simulink model "IMU_Filtering"  (R2021a)
settings: Solver=ode1  StartTime=0.0  StopTime=t_tot  FixedStep=T  RelTol=1e-3
values from neighbouring files (symbols this model uses):
  acc_init_matrix = [acc_init_matrix_1; acc_init_matrix_2]    [Main_Filtering.m]
  calibration_flag = calibration_flag+1    (= 1)    [Main_Filtering.m]
  chain_id_matrix = [little_chain ... (first row only)    [Main_Filtering.m]
  filter_par_vec = [beta, sample_f, max_acc_norm, min_acc_norm, gyro_th,                     n_imus, n_orientations, n_chains, n_phalanges]    [Main_Filtering.m]
  q_init_matrix = q_matrix.data(:,:,end)    [Main_Filtering.m]
  q_off_matrix = q_matrix.data(:,:,end)    [Main_Filtering.m]
undefined symbols (not defined in the file or in its folder): deg, s
libraries: CP_library x1, QB_pacer_lib x1, qbmove_library x1
settings Model: Creator=murad  LastModifiedBy=sohei
settings SolverCC: AlgebraicLoopSolver=TrustRegion
settings DataIOCC: ReturnWorkspaceOutputs=off
settings DebuggingCC: SFMachineParentedDataDiag=warning  ArithmeticOperatorsInVariantConditions=warning
settings SFSimCC: CustomCodeUndefinedFunction=UseInterfaceOnly

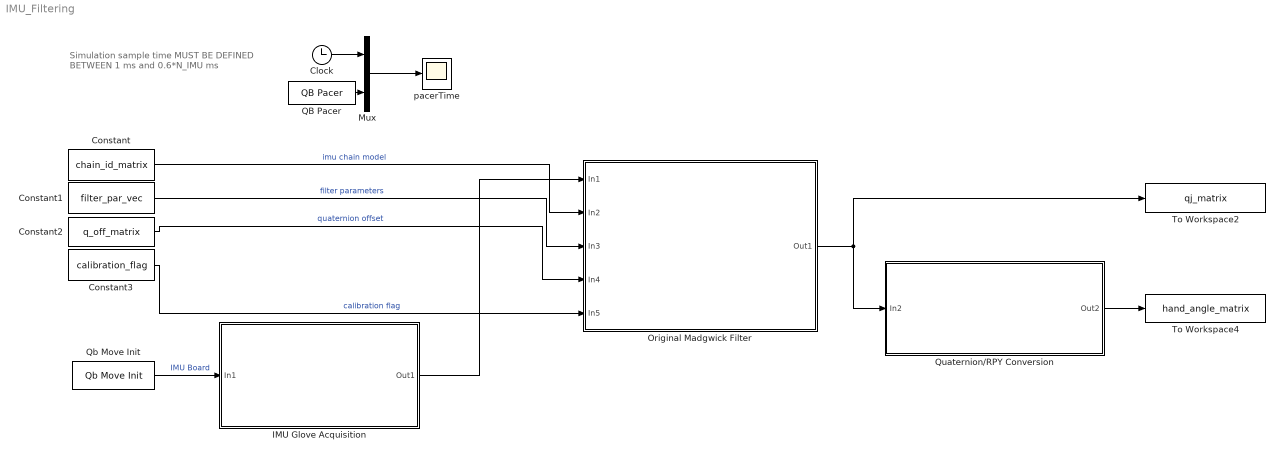
== system IMU_Filtering ==
  note: Simulation sample time
      | MUST BE DEFINED BETWEEN
      | 1 ms and 0.6*N_IMU ms
  Clock : Clock
  Constant : Constant  Value=chain_id_matrix
  Constant1 : Constant  Value=filter_par_vec
  Constant2 : Constant  Value=q_off_matrix
  Constant3 : Constant  Value=calibration_flag
  IMU Glove Acquisition : Subsystem
  Mux : Mux  Inputs=2
  Original Madgwick Filter : Subsystem
  QB Pacer : QB_pacer_lib/QB Pacer  simTimePerRealTime=1
      settings: SourceProductName=QB Pacer
  Qb Move Init : qbmove_library/Qb Move Init  NUMBER_OF_COM='COM3'  BAUD_RATE_COM=2000000
      settings: SourceProductName=Qb Move Library
  Quaternion/RPY Conversion : Subsystem
  To Workspace2 : ToWorkspace  VariableName=qj_matrix  SaveFormat=Timeseries  SampleTime=-1
  To Workspace4 : ToWorkspace  VariableName=hand_angle_matrix  SaveFormat=Timeseries  SampleTime=-1
  pacerTime : Scope
  wires:
  Mux/1 -> pacerTime/1
  QB Pacer/1 -> Mux/2
  Clock/1 -> Mux/1
  Qb Move Init/1 -> IMU Glove Acquisition/1(In1)  "IMU Board"
  IMU Glove Acquisition/1(Out1) -> Original Madgwick Filter/1(In1)
  Original Madgwick Filter/1(Out1) -> To Workspace2/1, Quaternion/RPY Conversion/1(In2)
  Quaternion/RPY Conversion/1(Out2) -> To Workspace4/1
  Constant/1 -> Original Madgwick Filter/2(In2)  "imu chain model"
  Constant1/1 -> Original Madgwick Filter/3(In3)  "filter parameters"
  Constant2/1 -> Original Madgwick Filter/4(In4)  "quaternion offset"
  Constant3/1 -> Original Madgwick Filter/5(In5)  "calibration flag"

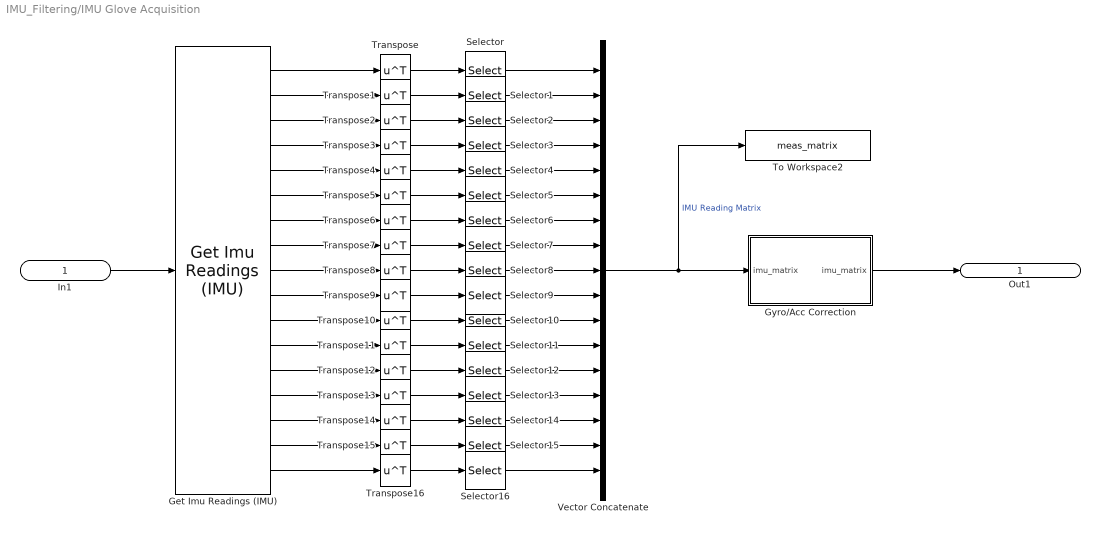
== system IMU_Filtering/IMU Glove Acquisition ==
  In1 : Inport
  Get Imu Readings (IMU) : CP_library/Get Imu Readings (IMU)  ID=3  N_IMU=17  DAISY_CHAINING=off  ACC_UNITY=G  GYRO_UNITY=deg/s  MAG_UNITY=uT
      settings: SourceProductName=Centro Piaggio Library
  Gyro/Acc Correction : MATLAB Function  TreatAsAtomicUnit=on
  Selector{,1..16} (17 alike) : Selector  InputPortWidth=14  IndexOptions=Index vector (dialog)  Indices=[1 2 3 4 5 6]  OutputSizes=1
  To Workspace2 : ToWorkspace  VariableName=meas_matrix  SaveFormat=Timeseries  SampleTime=-1
  Transpose{,1..16} (17 alike) : Math  Operator=transpose  SignedPower=on  SaturateOnIntegerOverflow=on
  Vector Concatenate : Concatenate  NumInputs=17  Mode=Multidimensional array  ConcatenateDimension=2
  Out1 : Outport  VectorParamsAs1DForOutWhenUnconnected=off
  wires:
  Get Imu Readings (IMU)/4 -> Transpose3/1
  Get Imu Readings (IMU)/3 -> Transpose2/1
  Transpose15/1 -> Selector15/1
  Transpose14/1 -> Selector14/1
  Transpose11/1 -> Selector11/1
  Get Imu Readings (IMU)/10 -> Transpose9/1
  Get Imu Readings (IMU)/8 -> Transpose7/1
  Get Imu Readings (IMU)/14 -> Transpose13/1
  Transpose7/1 -> Selector7/1
  Get Imu Readings (IMU)/7 -> Transpose6/1
  Transpose13/1 -> Selector13/1
  Get Imu Readings (IMU)/2 -> Transpose1/1
  Transpose6/1 -> Selector6/1
  In1/1 -> Get Imu Readings (IMU)/1
  Selector6/1 -> Vector Concatenate/7
  Selector4/1 -> Vector Concatenate/5
  Selector10/1 -> Vector Concatenate/11
  Transpose2/1 -> Selector2/1
  Selector9/1 -> Vector Concatenate/10
  Transpose9/1 -> Selector9/1
  Get Imu Readings (IMU)/13 -> Transpose12/1
  Selector5/1 -> Vector Concatenate/6
  Selector3/1 -> Vector Concatenate/4
  Get Imu Readings (IMU)/12 -> Transpose11/1
  Get Imu Readings (IMU)/16 -> Transpose15/1
  Get Imu Readings (IMU)/11 -> Transpose10/1
  Selector8/1 -> Vector Concatenate/9
  Get Imu Readings (IMU)/9 -> Transpose8/1
  Selector1/1 -> Vector Concatenate/2
  Transpose/1 -> Selector/1
  Get Imu Readings (IMU)/5 -> Transpose4/1
  Selector2/1 -> Vector Concatenate/3
  Selector14/1 -> Vector Concatenate/15
  Selector7/1 -> Vector Concatenate/8
  Transpose1/1 -> Selector1/1
  Get Imu Readings (IMU)/15 -> Transpose14/1
  Selector11/1 -> Vector Concatenate/12
  Get Imu Readings (IMU)/6 -> Transpose5/1
  Selector13/1 -> Vector Concatenate/14
  Selector16/1 -> Vector Concatenate/17
  Transpose5/1 -> Selector5/1
  Transpose3/1 -> Selector3/1
  Transpose10/1 -> Selector10/1
  Selector12/1 -> Vector Concatenate/13
  Selector15/1 -> Vector Concatenate/16
  Transpose4/1 -> Selector4/1
  Get Imu Readings (IMU)/17 -> Transpose16/1
  Transpose8/1 -> Selector8/1
  Selector/1 -> Vector Concatenate/1
  Get Imu Readings (IMU)/1 -> Transpose/1
  Vector Concatenate/1 -> To Workspace2/1, Gyro/Acc Correction/1("imu_matrix ")  "IMU Reading Matrix"
  Transpose16/1 -> Selector16/1
  Transpose12/1 -> Selector12/1
  Gyro/Acc Correction/1(imu_matrix) -> Out1/1

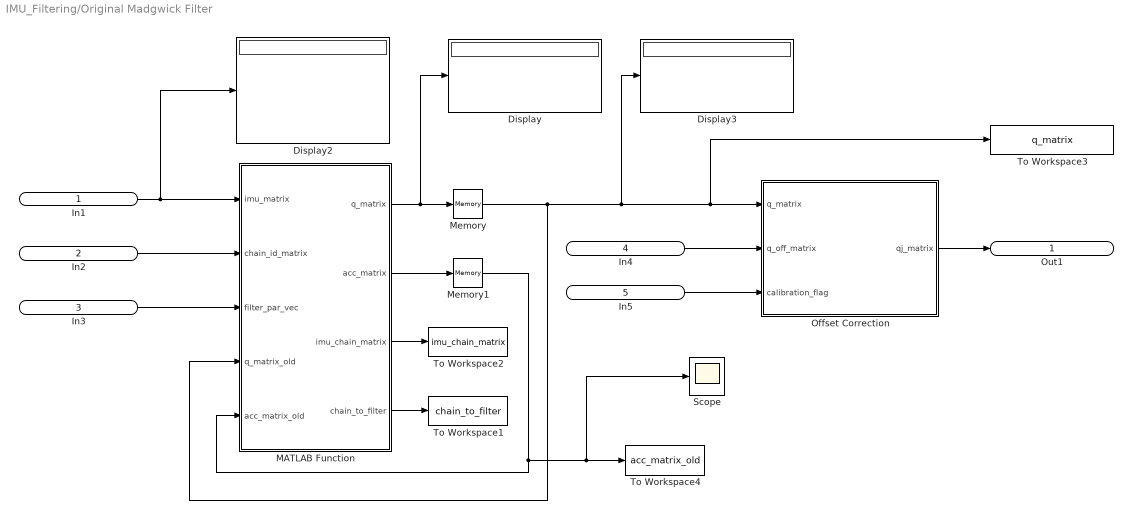
== system IMU_Filtering/Original Madgwick Filter ==
  In1 : Inport
  In2 : Inport  Port=2
  In3 : Inport  Port=3
  In4 : Inport  Port=4
  In5 : Inport  Port=5
  Display : Display
  Display2 : Display
  Display3 : Display
  MATLAB Function : MATLAB Function  TreatAsAtomicUnit=on
  Memory : Memory  InitialCondition=q_init_matrix  LinearizeAsDelay=on
  Memory1 : Memory  InitialCondition=acc_init_matrix  LinearizeAsDelay=on
  Offset Correction : MATLAB Function  TreatAsAtomicUnit=on
  Scope : Scope
  To Workspace1 : ToWorkspace  VariableName=chain_to_filter  SaveFormat=Timeseries  SampleTime=-1
  To Workspace2 : ToWorkspace  VariableName=imu_chain_matrix  SaveFormat=Timeseries  SampleTime=-1
  To Workspace3 : ToWorkspace  VariableName=q_matrix  SaveFormat=Timeseries  SampleTime=-1
  To Workspace4 : ToWorkspace  VariableName=acc_matrix_old  SaveFormat=Timeseries  SampleTime=-1
  Out1 : Outport  VectorParamsAs1DForOutWhenUnconnected=off
  wires:
  MATLAB Function/1(q_matrix) -> Memory/1, Display/1
  In1/1 -> Display2/1, MATLAB Function/1(imu_matrix)
  In2/1 -> MATLAB Function/2(chain_id_matrix)
  In3/1 -> MATLAB Function/3(filter_par_vec)
  Memory1/1 -> MATLAB Function/5(acc_matrix_old), Scope/1, To Workspace4/1
  MATLAB Function/2(acc_matrix) -> Memory1/1
  In4/1 -> Offset Correction/2(q_off_matrix)
  In5/1 -> Offset Correction/3(calibration_flag)
  Offset Correction/1(qj_matrix) -> Out1/1
  MATLAB Function/3(imu_chain_matrix) -> To Workspace2/1
  MATLAB Function/4(chain_to_filter) -> To Workspace1/1
  Memory/1 -> MATLAB Function/4(q_matrix_old), To Workspace3/1, Offset Correction/1(q_matrix), Display3/1

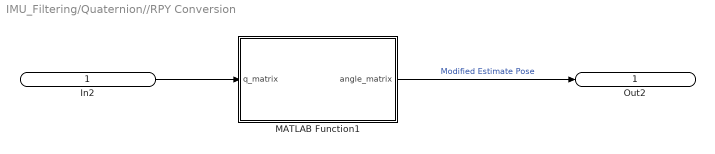
== system IMU_Filtering/Quaternion//RPY Conversion ==
  In2 : Inport
  MATLAB Function1 : MATLAB Function  TreatAsAtomicUnit=on
  Out2 : Outport  VectorParamsAs1DForOutWhenUnconnected=off
  wires:
  In2/1 -> MATLAB Function1/1(q_matrix)
  MATLAB Function1/1(angle_matrix) -> Out2/1  "Modified Estimate Pose"

== matlab function IMU_Filtering/Original Madgwick Filter/MATLAB Function ==
  data: imu_matrix input; chain_id_matrix input; filter_par_vec input; q_matrix_old input; acc_matrix_old input; q_matrix output; acc_matrix output; imu_chain_matrix output; chain_to_filter output
function [q_matrix, acc_matrix, imu_chain_matrix, chain_to_filter]  = ...
        Filtering_Process(imu_matrix, chain_id_matrix, filter_par_vec, ...
        q_matrix_old, acc_matrix_old)

% IMU chain definitions
%imu_chain_matrix = glove_start(imu_matrix, filter_param_struct);

% IMU chain matrix definition (see the config.yaml file)
% The imus are arranged as:
% columns 1-4 -> little chain (ids: 2 1 0 15)
% columns 5-8 -> ring chain (ids: 5 4 3 15)
% columns 9-12 -> medium chain (ids: 8 7 6 15)
% columns 13-16 -> chain (ids: 11 10 9 15)
% columns 17-24 -> thumb chain (ids: 14 13 12 16)
% IMU ids are contained in matrix first row (each one plus 1)
% subsequent rows contain accelerometer and gyro readings

gyro_th = filter_par_vec(5);

cont = 0;
imu_chain_matrix = zeros(7,20);

for i = 1:5
    for k = 1:4 
        for j = 1:17
            if j == chain_id_matrix(i,k)
                cont = cont+1;
                imu_chain_matrix(1,cont)    = j;
                imu_chain_matrix(2:7,cont)  = imu_matrix(:,j);
            end
        end
    end
end

% Quaternion estimate computation from IMU readings via the Madgwick filter

cont            = 0;
q_matrix        = zeros(4,15);
acc_matrix      = zeros(3,20);
chain_to_filter = zeros(2,15);

for i = 1:5 % number of imu chains
    
    for j = 1:3 % number of phalanges
        
        cont = cont+1;
        
        % Definition of the two imus on which the filter is applied;
        % the filter computes the quaternion representing the relative
        % orientation between imu_world and imu_sensor, expressed in the
        % imu_world frame
        imu_sensor  = imu_chain_matrix(:,4*(i-1)+j);
        imu_world   = imu_chain_matrix(:,4*(i-1)+j+1); 
        
        % Filtering the gyroscope (see IMUGL::InitialOffset and
        % IMUGL::computeAngles)
            
        for k = 1:3

            if abs(imu_sensor(4+k)) < gyro_th
                imu_sensor(4+k) = 0;
            end

            if abs(imu_world(4+k)) < gyro_th
                imu_world(4+k) = 0;
            end
            
        end
        
        
        % Verify the two imus passed to the filter
        chain_to_filter(1,cont) = imu_sensor(1)-1;
        chain_to_filter(2,cont) = imu_world(1)-1;
        
        qL_old      = q_matrix_old(:,cont);
        
        aP_old      = acc_matrix_old(:,4*(i-1)+j);
        aN_old      = acc_matrix_old(:,4*(i-1)+j+1);
        
        [qL, aP, aN] = my_Madgwick_Filter(imu_sensor, imu_world, qL_old, ...
                                            aP_old, aN_old, filter_par_vec);                               
        q_matrix(:,cont) = qL;
        
        acc_matrix(:,4*(i-1)+j)     = aP;
        acc_matrix(:,4*(i-1)+j+1)   = aN;
                                           
    end
    
    % At the end of the filtering process I obtain a matrix 4*15, where
    % every quaternion for each imu pair is contained
    
end

== matlab function IMU_Filtering/Original Madgwick Filter/Offset Correction ==
  data: q_matrix input; qj_matrix output; q_off_matrix input; calibration_flag input
function qj_matrix = offset_correction(q_matrix, q_off_matrix, calibration_flag)

persistent off_cont;
qj_matrix = zeros(size(q_matrix,1),size(q_matrix,2));

if isempty(off_cont)
        off_cont = 0;
end

if calibration_flag == 2
    
    for i = 1:15
        
        q       = q_matrix(:,i);
        qoff    = q_off_matrix(:,i);
        
        qj_matrix(:,i) =  [ qoff(1)*q(1) + qoff(2)*q(2) + qoff(3)*q(3) + qoff(4)*q(4);
                            qoff(1)*q(2) - qoff(2)*q(1) - qoff(3)*q(4) + qoff(4)*q(3);
                            qoff(1)*q(3) - qoff(3)*q(1) - qoff(4)*q(2) + qoff(2)*q(4);
                            qoff(1)*q(4) - qoff(4)*q(1) - qoff(2)*q(3) + qoff(3)*q(2)];      
    end

else
    qj_matrix = q_matrix;
    off_cont = off_cont + 1;
    %disp(off_cont)
end
    
end

== matlab function IMU_Filtering/IMU Glove Acquisition/Gyro//Acc Correction ==
  data: imu_matrix input; imu_matrix output
function imu_matrix = gyro_acc_correction(imu_matrix)

% correction of gyro and accelerometer readings for imus 1, 4, 7, 10 and 13
% (see IMUGL:callbackAcc and IMUGL:callbackGyro)

for i = 1:17
    if i == 2 || i == 5 || i == 8 || i == 11 || i == 14
        
        % accelerometer, x and y
        imu_matrix(1,i) = -imu_matrix(1,i);
        imu_matrix(2,i) = -imu_matrix(2,i);

        % gyroscope, x and y
        imu_matrix(4,i) = -imu_matrix(4,i);
        imu_matrix(5,i) = -imu_matrix(5,i);  
        
    end
end

== matlab function IMU_Filtering/Quaternion//RPY Conversion/MATLAB Function1 ==
  data: q_matrix input; angle_matrix output

function angle_matrix = quat_to_rpy(q_matrix)

% RPY angle computation from Madgwick filter quaternions (in degrees)

angle_matrix = zeros(3,15);

for i = 1:15
    
    w = q_matrix(1,i);
    x = q_matrix(2,i);
    y = q_matrix(3,i);
    z = q_matrix(4,i);
    
    angle_matrix(1,i) = asin(2*x*z + 2*w*y)*180/pi;                    % Roll angle
    angle_matrix(2,i) = atan2(2*y*z - 2*w*x, 2*w*w + 2*z*z - 1)*180/pi; % Pitch angle
    angle_matrix(3,i) = atan2(2*x*y - 2*w*z, 2*w*w + 2*x*x - 1)*180/pi; % Yaw angle
    
end
